simulink model "Robot_Oystein_HOG"  (R2019b)
settings: Solver=VariableStepAuto  StartTime=0.0  StopTime=10.0  RelTol=1e-5  EnableMultiTasking=on
model workspace (MATLAB code in the model file):
  | g=9.81;
  | L1=0.240;
  | L2=0.800;
  | L3=1.050;
  | L4=1.175;
  | L5=0.225;
  | L6=0.200;
  | L7=0.235;
  | L8=0.248;
  | L_BC=0.300;
  | W_BC=0.05;
  | L_BD=0.400;
  | W_BE=W_BC;
  | L_EF=0.400;
  | L_EG=0.225;
  | L_GH=1.175;
  | L_HI=0.200;
  | L_IJ=0.235;
  | H_IJ=0.248;
undefined symbols (not defined in the file): X, Y, Z
libraries: sm_lib x46, nesl_utility x4
(part 2 of 2)

== matlab function Robot_Oystein_HOG/MATLAB Function ==
  data: x output; t input; y output; z output
function [x,y,z] = fcn(t)
A=0.2;
x=1.6;
y=0.0;
z=0.9;
end
